simulink model "uav_trim_va_h_chi_sim"  (R2024a)
settings: Solver=ode45  StartTime=0.0  StopTime=36e1  FixedStep=0.1  RelTol=1e-3
values from neighbouring files (symbols this model uses):
  uavParams = make_uav_parameters_eimpc()    [main_sim_eimpc.m]    (also in main_sim_pid.m; make_uav_parameters_eimpc.m = NaN(60,1))
undefined symbols (not defined in the file or in its folder): gamma_trim
settings Model: Creator=pf  LastModifiedBy=piotr
settings RTWCC: GPUComputeCapability=3.5

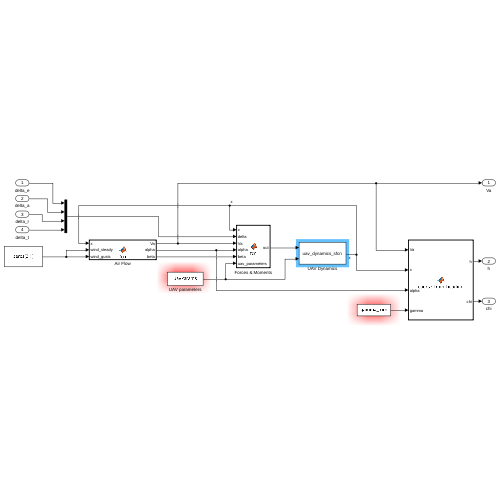
[thumbnail: Simulink's stored preview of the top-level diagram]
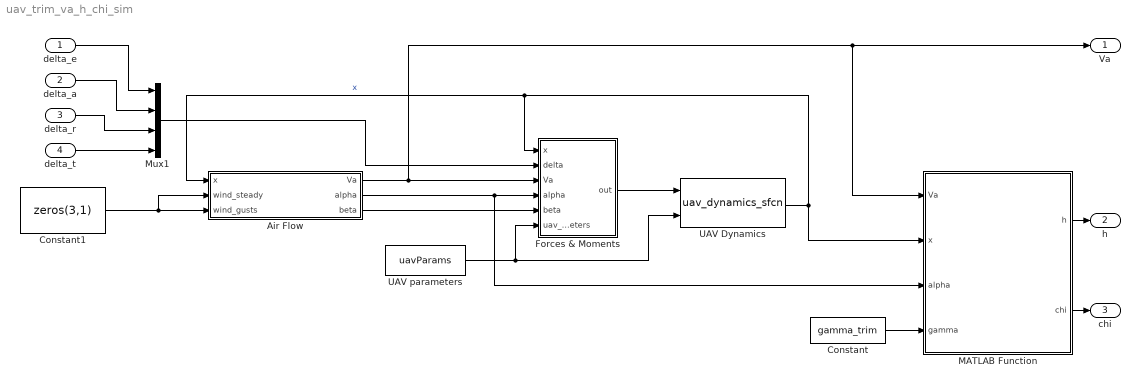
== system uav_trim_va_h_chi_sim ==
  delta_e : Inport
  delta_a : Inport  Port=2
  delta_r : Inport  Port=3
  delta_t : Inport  Port=4
  Air Flow : MATLAB Function  TreatAsAtomicUnit=on
  Constant : Constant  Value=gamma_trim
  Constant1 : Constant  Value=zeros(3,1)
  Forces & Moments : MATLAB Function  TreatAsAtomicUnit=on
  MATLAB Function : MATLAB Function  TreatAsAtomicUnit=on
  Mux1 : Mux
  UAV Dynamics : M-S-Function  FunctionName=uav_dynamics_sfcn  Parameters=x0
  UAV parameters : Constant  Value=uavParams
  Va : Outport
  h : Outport  Port=2
  chi : Outport  Port=3
  wires:
  UAV Dynamics/1 -> Air Flow/1(x), Forces & Moments/1(x), MATLAB Function/2(x)  "x"
  delta_e/1 -> Mux1/1
  delta_a/1 -> Mux1/2
  delta_r/1 -> Mux1/3
  delta_t/1 -> Mux1/4
  MATLAB Function/2(chi) -> chi/1
  Constant/1 -> MATLAB Function/4(gamma)
  Air Flow/1(Va) -> MATLAB Function/1(Va), Va/1, Forces & Moments/3(Va)
  Air Flow/2(alpha) -> MATLAB Function/3(alpha), Forces & Moments/4(alpha)
  Air Flow/3(beta) -> Forces & Moments/5(beta)
  UAV parameters/1 -> UAV Dynamics/2, Forces & Moments/6(uav_parameters)
  Mux1/1 -> Forces & Moments/2(delta)
  Forces & Moments/1(out) -> UAV Dynamics/1
  MATLAB Function/1(h) -> h/1
  Constant1/1 -> Air Flow/3(wind_gusts), Air Flow/2(wind_steady)

== matlab function uav_trim_va_h_chi_sim/Forces & Moments ==
  data: x input; out output; delta input; Va input; alpha input; beta input; uav_parameters input
function out = fcn(x, delta, Va, alpha, beta, uav_parameters)
    out = forces_moments(x, delta, Va, alpha, beta, uav_parameters);
end

== matlab function uav_trim_va_h_chi_sim/MATLAB Function ==
  data: Va input; h output; x input; alpha input; chi output; gamma input
function [h,chi] = course_from_heading(Va,x,alpha,gamma)
    % chi - course
    % Va - airspeed
    % uvw = [u;v;w] - components of ground speed
    % theta - pitch, rad
    % psi - heading, rad
    % alpha - angle of attack, rad
    % gamma - flight path angle, rad
    % we - wind in East direction
    h = -x(3);
    uvw = x(4:6);
    theta   = x(8); % pitch angle
    psi     = x(9); % yaw angle
    we = 0;
    sinchi = (Va*sin(psi)*cos(theta-alpha)+we) / (norm(uvw)*cos(gamma));
    chi = asin(sinchi);
end

== matlab function uav_trim_va_h_chi_sim/Air Flow ==
  data: x input; Va output; wind_steady input; wind_gusts input; alpha output; beta output
function [Va, alpha, beta] = fcn(x,wind_steady,wind_gusts)
    [Va, alpha, beta] = airdata(x,wind_steady,wind_gusts);
end
